simulink model "Integration_Forward_Forger_L"  (R2015a)
settings: Solver=ode3  StartTime=0.0  StopTime=400  FixedStep=0.01  MaxStep=0.01  RelTol=1e-3
values from neighbouring files (symbols this model uses):
  I_update = I    [Gradient_Descent_Greedy_3rd.m]
  n0 = Periodic_Solution(time_shift(j)*100+1,4)    [Gradient_Descent_Greedy_3rd.m]
  Periodic_Solution = Periodic_Solution(101:end,:)    [Gradient_Descent_Greedy_3rd.m]    (also in Periodic_Solution_JFK_1000lux.mat = [0 0.00999999999999 0.02 0.03 0.04 0.05 0.0599999999999 0.06)
  T_opt = x(end,1)    [Gradient_Descent_Greedy_3rd.m]
  tol = 0.01    [Gradient_Descent_Greedy_3rd.m]
  x0 = Periodic_Solution(time_shift(j)*100+1,2)    [Gradient_Descent_Greedy_3rd.m]
  xc0 = Periodic_Solution(time_shift(j)*100+1,3)    [Gradient_Descent_Greedy_3rd.m]
settings Model: Creator=wangf7  LastModifiedBy=Jiawei Yin
settings OptimizationCC: ExpressionDepthLimit=2147483647
settings DebuggingCC: UnderspecifiedInitializationDetection=Classic  MergeDetectMultiDrivingBlocksExec=none  SolverPrmCheckMsg=warning  StateNameClashWarn=warning

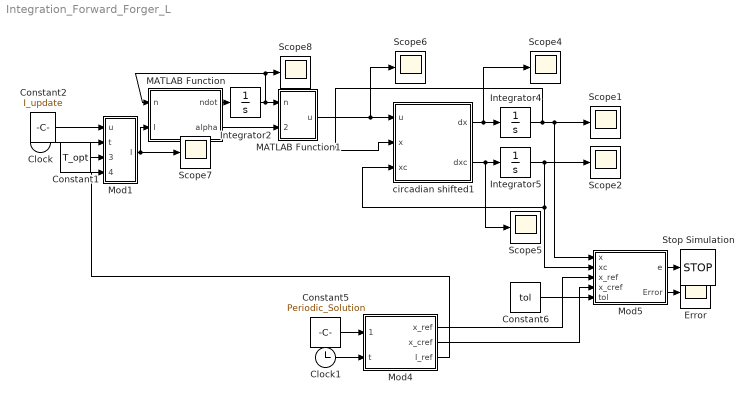
== system Integration_Forward_Forger_L ==
  Clock : Clock
  Clock1 : Clock
  Constant1 : Constant  Value=T_opt
  Constant2 : Constant  Value=I_update
  Constant5 : Constant  Value=Periodic_Solution
  Constant6 : Constant  Value=tol
  Error : Scope
      settings: TimeRange=auto  MaxDataPoints=50000000  SaveName=Error  YMin=-0.55525  YMax=5.16915  SampleTime=-1  DataFormat=Array
  Integrator2 : Integrator  InitialCondition=n0
  Integrator4 : Integrator  InitialCondition=x0
  Integrator5 : Integrator  InitialCondition=xc0
  MATLAB Function : MATLAB Function  TreatAsAtomicUnit=on
      settings: PermitHierarchicalResolution=ParametersOnly
  MATLAB Function1 : MATLAB Function  TreatAsAtomicUnit=on
      settings: PermitHierarchicalResolution=ParametersOnly
  Mod1 : MATLAB Function  TreatAsAtomicUnit=on
      settings: PermitHierarchicalResolution=ParametersOnly
  Mod4 : MATLAB Function  TreatAsAtomicUnit=on
      settings: PermitHierarchicalResolution=ParametersOnly
  Mod5 : MATLAB Function  TreatAsAtomicUnit=on
      settings: PermitHierarchicalResolution=ParametersOnly
  Scope{1..2,4..8} (7 alike) : Scope
      Scope1 settings: TimeRange=auto  MaxDataPoints=50000000  SaveName=x  YMin=-1.34782  YMax=1.30409  SampleTime=-1  DataFormat=Array
      Scope2 settings: TimeRange=auto  MaxDataPoints=50000000  SaveName=xc  YMin=-1.44853  YMax=1.30585  SampleTime=-1  DataFormat=Array
      Scope4 settings: TimeRange=auto  MaxDataPoints=50000000  SaveName=dx  YMin=-0.12715  YMax=0.13151  SampleTime=-1  DataFormat=Array
      Scope5 settings: TimeRange=auto  MaxDataPoints=50000000  SaveName=dxc  YMin=-0.12715  YMax=0.13151  SampleTime=-1  DataFormat=Array
      Scope6 settings: TimeRange=auto  MaxDataPoints=50000000  SaveName=u  YMin=-0.12715  YMax=0.13151  SampleTime=-1  DataFormat=Array
      Scope7 settings: TimeRange=auto  MaxDataPoints=50000000  SaveName=I  YMin=-0.12715  YMax=0.13151  SampleTime=-1  DataFormat=Array
      Scope8 settings: TimeRange=auto  MaxDataPoints=50000000  SaveName=n  YMin=-0.12715  YMax=0.13151  SampleTime=-1  DataFormat=Array
  Stop Simulation : Stop
  circadian shifted1 : MATLAB Function  TreatAsAtomicUnit=on
      settings: PermitHierarchicalResolution=ParametersOnly
  wires:
  circadian shifted1/1(dx) -> Scope4/1, Integrator4/1
  circadian shifted1/2(dxc) -> Scope5/1, Integrator5/1
  Integrator4/1 -> circadian shifted1/2(x), Mod5/1(x), Scope1/1
  Clock/1 -> Mod1/2(t)
  Constant2/1 -> Mod1/1(u)
  Integrator5/1 -> Mod5/2(xc), circadian shifted1/3(xc), Scope2/1
  Constant5/1 -> Mod4/1(Periodic_Solution)
  Clock1/1 -> Mod4/2(t)
  Mod5/1(e) -> Stop Simulation/1
  Mod4/1(x_ref) -> Mod5/3(x_ref)
  Mod4/2(x_cref) -> Mod5/4(x_cref)
  Constant6/1 -> Mod5/5(tol)
  Constant1/1 -> Mod1/3(T_opt)
  MATLAB Function/1(ndot) -> Integrator2/1
  Integrator2/1 -> Scope8/1, MATLAB Function/1(n), MATLAB Function1/1(n)
  MATLAB Function/2(alpha) -> MATLAB Function1/2(alpha)
  Mod1/1(I) -> MATLAB Function/2(I), Scope7/1
  MATLAB Function1/1(u) -> Scope6/1, circadian shifted1/1(u)
  Mod4/3(I_ref) -> Mod1/4(Iref)
  Mod5/2(Error) -> Error/1

== matlab function Integration_Forward_Forger_L/MATLAB Function ==
  data: n input; I input; ndot output; alpha output
function [ndot,alpha] = fcn(n,I)

alpha0=0.05;
beta=0.0075;
I0=9500;
alpha=alpha0*(I/I0)^0.5;
ndot=60*[alpha*(1-n)-beta*n];

== matlab function Integration_Forward_Forger_L/Mod1 ==
  data: u input; I output; t input; T_opt input; Iref input
function I  = fcn(u,t,T_opt,Iref)
%#codegen
if t==0
    I=u(1,2);
elseif t<=T_opt
    I=interp1q(u(:,1),u(:,2),t);
else
    I=Iref;
end

== matlab function Integration_Forward_Forger_L/circadian shifted1 ==
  data: u input; x input; xc input; dx output; dxc output
function [dx,dxc] = fcn(u,x,xc)

k=0.55;
mu=0.13;
q=1/3;
B=(1-0.4*x)*(1-0.4*xc)*u;
tau=24.2;

dx = pi*(xc+mu*(x/3+4*x^3/3-256*x^7/105)+B)/12;
dxc = pi*(q*B*xc-x*((24/0.99729/tau)^2+k*B))/12;

== matlab function Integration_Forward_Forger_L/Mod4 ==
  data: Periodic_Solution input; x_ref output; t input; x_cref output; I_ref output
function [x_ref,x_cref,I_ref] = fcn(Periodic_Solution,t)
%#codegen
x_ref=interp1q(Periodic_Solution(:,1),Periodic_Solution(:,2),t);
x_cref=interp1q(Periodic_Solution(:,1),Periodic_Solution(:,3),t);
I_ref=interp1q(Periodic_Solution(:,1),Periodic_Solution(:,6),t);

== matlab function Integration_Forward_Forger_L/Mod5 ==
  data: x input; xc input; e output; x_ref input; x_cref input; tol input; Error output
function [e,Error] = fcn(x,xc,x_ref,x_cref,tol)
%#codege
Error=(x-x_ref)^2+(xc-x_cref)^2;
e=Error<tol;

== matlab function Integration_Forward_Forger_L/MATLAB Function1 ==
  data: n input; u output; alpha input
function u = fcn(n,alpha)
%#codegen
u=33.75*alpha*(1-n);
